simulink library "surfaceCoefficients_ul"  (R2018b)
settings: Solver=VariableStepAuto  StartTime=0.0  StopTime=10.0  RelTol=1e-3
settings Model: Creator=mcobb  LastModifiedBy=mcobb

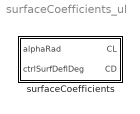
== system surfaceCoefficients_ul ==
  surfaceCoefficients : Subsystem

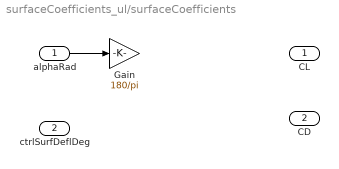
== system surfaceCoefficients_ul/surfaceCoefficients ==
  alphaRad : Inport
  ctrlSurfDeflDeg : Inport  Port=2
  Gain : Gain  Gain=180/pi
  CL : Outport
  CD : Outport  Port=2
  wires:
  alphaRad/1 -> Gain/1
